simulink model "InvertedPendulum_sim"  (R2019a)
settings: Solver=ode113  StartTime=0.0  StopTime=100  RelTol=1e-3
settings Model: Creator=黄原  LastModifiedBy=黄原

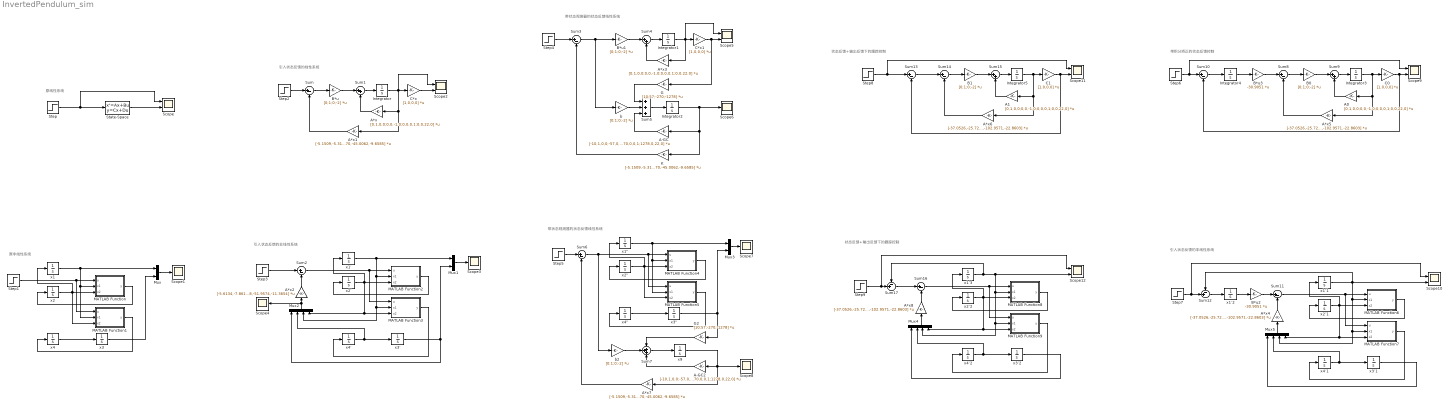
== system InvertedPendulum_sim ==
  note: 原非线性系统
  note: 原线性系统
  note: 引入状态反馈的线性系统
  note: 引入状态反馈的非线性系统
  note: 带状态观测器的状态反馈线性系统
  note: 带状态观测器的状态反馈线性系统
  note: 带积分矫正的状态反馈控制
  note: 引入状态反馈的非线性系统
  note: 状态反馈+输出反馈下的跟踪控制
  note: 状态反馈+输出反馈下的跟踪控制
  A*x : Gain  Gain=[0,1,0,0;0,0,-1,0;0,0,0,1;0,0,22,0]  Multiplication=Matrix(K*u)
  A*x1 : Gain  Gain=[-5.1509,-5.3170,-45.0062,-9.6585]  Multiplication=Matrix(K*u)
  A*x2 : Gain  Gain=[-5.6134,-7.8618,-51.9574,-11.3654]  Multiplication=Matrix(K*u)
  A*x3 : Gain  Gain=[0,1,0,0;0,0,-1,0;0,0,0,1;0,0,22,0]  Multiplication=Matrix(K*u)
  A*x{4..6,8} (4 alike) : Gain  Gain=[-37.0526,-25.7207,-102.9571,-22.8603]  Multiplication=Matrix(K*u)
  A*x7 : Gain  Gain=[-5.1509,-5.3170,-45.0062,-9.6585]  Multiplication=Matrix(K*u)
  A-GC : Gain  Gain=[-10,1,0,0;-57,0,-1,0;270,0,0,1;1278,0,22,0]  Multiplication=Matrix(K*u)
  A-GC2 : Gain  Gain=[-10,1,0,0;-57,0,-1,0;270,0,0,1;1278,0,22,0]  Multiplication=Matrix(K*u)
  A0 : Gain  Gain=[0,1,0,0;0,0,-1,0;0,0,0,1;0,0,22,0]  Multiplication=Matrix(K*u)
  A1 : Gain  Gain=[0,1,0,0;0,0,-1,0;0,0,0,1;0,0,22,0]  Multiplication=Matrix(K*u)
  B*u : Gain  Gain=[0;1;0;-2]  Multiplication=Matrix(K*u)
  B*u1 : Gain  Gain=[0;1;0;-2]  Multiplication=Matrix(K*u)
  B*u2 : Gain  Gain=-30.9051  Multiplication=Matrix(K*u)
  B*u3 : Gain  Gain=-30.9051  Multiplication=Matrix(K*u)
  B0 : Gain  Gain=[0;1;0;-2]  Multiplication=Matrix(K*u)
  B1 : Gain  Gain=[0;1;0;-2]  Multiplication=Matrix(K*u)
  C*x : Gain  Gain=[1,0,0,0]  Multiplication=Matrix(K*u)
  C*x1 : Gain  Gain=[1,0,0,0]  Multiplication=Matrix(K*u)
  C0 : Gain  Gain=[1,0,0,0]  Multiplication=Matrix(K*u)
  C1 : Gain  Gain=[1,0,0,0]  Multiplication=Matrix(K*u)
  G : Gain  Gain=[10;57;-270;-1278]  Multiplication=Matrix(K*u)
  G2 : Gain  Gain=[10;57;-270;-1278]  Multiplication=Matrix(K*u)
  Integrator{,1..2,5} (4 alike) : Integrator  InitialCondition=[0.1,0.1,0.1,0.1]
  Integrator3 : Integrator  InitialCondition=[0,0,0,0]
  Integrator4 : Integrator
  K : Gain  Gain=[-5.1509,-5.3170,-45.0062,-9.6585]  Multiplication=Matrix(K*u)
  MATLAB Function : MATLAB Function  TreatAsAtomicUnit=on
  MATLAB Function1 : MATLAB Function  TreatAsAtomicUnit=on
  MATLAB Function2 : MATLAB Function  TreatAsAtomicUnit=on
  MATLAB Function3 : MATLAB Function  TreatAsAtomicUnit=on
  MATLAB Function4 : MATLAB Function  TreatAsAtomicUnit=on
  MATLAB Function5 : MATLAB Function  TreatAsAtomicUnit=on
  MATLAB Function6 : MATLAB Function  TreatAsAtomicUnit=on
  MATLAB Function7 : MATLAB Function  TreatAsAtomicUnit=on
  MATLAB Function8 : MATLAB Function  TreatAsAtomicUnit=on
  MATLAB Function9 : MATLAB Function  TreatAsAtomicUnit=on
  Mux : Mux  Inputs=2
  Mux1 : Mux  Inputs=2
  Mux2 : Mux
  Mux3 : Mux  Inputs=2
  Mux4 : Mux
  Mux5 : Mux
  Scope{,2,5,9..12} (7 alike) : Scope  NumInputPorts=2
  Scope{1,3..4,6..8} (6 alike) : Scope
  State-Space : StateSpace  A=[0,1,0,0;0,0,-1,0;0,0,0,1;0,0,22,0]  B=[0;1;0;-2]  C=[1,0,0,0]  D=0  InitialCondition=[0.1;0.1;0.1;0.1]
  Step{,1..5} (6 alike) : Step  After=0.01  SampleTime=0
  Step6 : Step  Time=3  SampleTime=0
  Step7 : Step  After=0.05  SampleTime=0
  Step8 : Step  After=0.05  SampleTime=0
  Step9 : Step  After=0.05  SampleTime=0
  Sum{,2..3,6,8,10..11,13..14,16} (10 alike) : Sum  Inputs=|+-
  Sum{1,4,9,15} (4 alike) : Sum  Inputs=|++
  Sum12 : Sum  Inputs=-+|
  Sum17 : Sum  Inputs=-+|
  Sum5 : Sum  Inputs=+++
  Sum7 : Sum  Inputs=+++
  b : Gain  Gain=[0;1;0;-2]  Multiplication=Matrix(K*u)
  b2 : Gain  Gain=[0;1;0;-2]  Multiplication=Matrix(K*u)
  x{1..4,9} (5 alike) : Integrator  InitialCondition=0.1
  x1'' : Integrator  InitialCondition=0.1
  x1‘ : Integrator  InitialCondition=0.1
  x1‘1 : Integrator  InitialCondition=0.1
  x1‘2 : Integrator
  x1‘3 : Integrator  InitialCondition=0.1
  "x2'' " : Integrator  InitialCondition=0.1
  x2’ : Integrator  InitialCondition=0.1
  x2’1 : Integrator  InitialCondition=0.1
  x2’2 : Integrator  InitialCondition=0.1
  x3'' : Integrator  InitialCondition=0.1
  x3’ : Integrator  InitialCondition=0.1
  x3’1 : Integrator  InitialCondition=0.1
  x3’2 : Integrator  InitialCondition=0.1
  x4'' : Integrator  InitialCondition=0.1
  x4‘ : Integrator  InitialCondition=0.1
  x4‘1 : Integrator  InitialCondition=0.1
  x4‘2 : Integrator  InitialCondition=0.1
  wires:
  x1/1 -> MATLAB Function1/2(x1), MATLAB Function/2(x1), Mux/1
  x2/1 -> x1/1, MATLAB Function/3(x2), MATLAB Function1/3(x2)
  MATLAB Function/1(y) -> x2/1
  x4/1 -> x3/1
  MATLAB Function1/1(y) -> x4/1
  Mux/1 -> Scope1/1
  x3/1 -> Mux/2
  State-Space/1 -> Scope/2
  Step1/1 -> MATLAB Function1/1(u), MATLAB Function/1(u)
  Step/1 -> State-Space/1, Scope/1
  Step2/1 -> Sum/1
  Sum/1 -> B*u/1
  B*u/1 -> Sum1/1
  Sum1/1 -> Integrator/1
  A*x/1 -> Sum1/2
  Integrator/1 -> A*x1/1, A*x/1, Scope2/1, C*x/1
  C*x/1 -> Scope2/2
  A*x1/1 -> Sum/2
  x1‘/1 -> Mux2/3, MATLAB Function3/2(x1), MATLAB Function2/2(x1), Mux1/1
  MATLAB Function2/1(y) -> x2’/1
  x2’/1 -> MATLAB Function2/3(x2), x1‘/1, Mux2/4, MATLAB Function3/3(x2)
  MATLAB Function3/1(y) -> x4‘/1
  Mux1/1 -> Scope3/1
  x3’/1 -> Mux1/2, Mux2/1
  x4‘/1 -> Mux2/2, x3’/1
  Step3/1 -> Sum2/1
  Sum2/1 -> MATLAB Function2/1(u), MATLAB Function3/1(u)
  A*x2/1 -> Sum2/2
  Mux2/1 -> Scope4/1, A*x2/1
  C*x1/1 -> G/1, Scope5/2
  Sum3/1 -> b/1, B*u1/1
  Sum4/1 -> Integrator1/1
  Integrator1/1 -> A*x3/1, Scope5/1, C*x1/1
  B*u1/1 -> Sum4/1
  Step4/1 -> Sum3/1
  A*x3/1 -> Sum4/2
  b/1 -> Sum5/2
  G/1 -> Sum5/1
  Sum5/1 -> Integrator2/1
  Integrator2/1 -> K/1, A-GC/1, Scope6/1
  A-GC/1 -> Sum5/3
  K/1 -> Sum3/2
  x1''/1 -> MATLAB Function5/2(x1), MATLAB Function4/2(x1), Mux3/1
  MATLAB Function4/1(y) -> "x2'' "/1
  "x2'' "/1 -> x1''/1, MATLAB Function4/3(x2), MATLAB Function5/3(x2)
  MATLAB Function5/1(y) -> x4''/1
  Mux3/1 -> Scope7/1
  x3''/1 -> G2/1, Mux3/2
  x4''/1 -> x3''/1
  Step5/1 -> Sum6/1
  Sum6/1 -> MATLAB Function5/1(u), MATLAB Function4/1(u), b2/1
  b2/1 -> Sum7/2
  Sum7/1 -> x9/1
  G2/1 -> Sum7/1
  A-GC2/1 -> Sum7/3
  x9/1 -> Scope8/1, A*x7/1, A-GC2/1
  A*x7/1 -> Sum6/2
  C0/1 -> Sum10/2, Scope9/2
  Sum8/1 -> B0/1
  A*x5/1 -> Sum8/2
  Sum9/1 -> Integrator3/1
  Integrator3/1 -> A*x5/1, A0/1, C0/1
  B0/1 -> Sum9/1
  A0/1 -> Sum9/2
  B*u3/1 -> Sum8/1
  Integrator4/1 -> B*u3/1
  Sum10/1 -> Integrator4/1
  Step6/1 -> Sum10/1, Scope9/1
  Sum11/1 -> MATLAB Function6/1(u), MATLAB Function7/1(u)
  A*x4/1 -> Sum11/2
  x4‘1/1 -> Mux5/2, x3’1/1
  x3’1/1 -> Mux5/1
  x1‘1/1 -> Scope10/2, Sum12/1, Mux5/3, MATLAB Function7/2(x1), MATLAB Function6/2(x1)
  MATLAB Function6/1(y) -> x2’1/1
  x2’1/1 -> MATLAB Function6/3(x2), x1‘1/1, Mux5/4, MATLAB Function7/3(x2)
  Mux5/1 -> A*x4/1
  MATLAB Function7/1(y) -> x4‘1/1
  Step7/1 -> Sum12/2, Scope10/1
  Sum12/1 -> x1‘2/1
  x1‘2/1 -> B*u2/1
  B*u2/1 -> Sum11/1
  Sum13/1 -> Sum14/1
  A1/1 -> Sum15/2
  Integrator5/1 -> A*x6/1, A1/1, C1/1
  C1/1 -> Sum13/2, Scope11/2
  Sum14/1 -> B1/1
  B1/1 -> Sum15/1
  Sum15/1 -> Integrator5/1
  Step8/1 -> Sum13/1, Scope11/1
  A*x6/1 -> Sum14/2
  Sum17/1 -> Sum16/1
  Mux4/1 -> A*x8/1
  MATLAB Function9/1(y) -> x4‘2/1
  x2’2/1 -> MATLAB Function8/3(x2), x1‘3/1, Mux4/4, MATLAB Function9/3(x2)
  x1‘3/1 -> Scope12/2, Mux4/3, MATLAB Function9/2(x1), MATLAB Function8/2(x1), Sum17/1
  MATLAB Function8/1(y) -> x2’2/1
  x4‘2/1 -> Mux4/2, x3’2/1
  x3’2/1 -> Mux4/1
  A*x8/1 -> Sum16/2
  Step9/1 -> Scope12/1, Sum17/2
  Sum16/1 -> MATLAB Function8/1(u), MATLAB Function9/1(u)

== matlab function InvertedPendulum_sim/MATLAB Function1 ==
  data: u input; y output; x1 input; x2 input
function y = fcn(u,x1,x2)

y = (u+0.05*sin(x1*x2*x2)-cos(x1)*sin(x1))/(1.1-0.1*cos(x1)*cos(x1));

== matlab function InvertedPendulum_sim/MATLAB Function ==
  data: u input; y output; x1 input; x2 input
function y = fcn(u,x1,x2)

y = (u*cos(x1)-11*sin(x1)+0.05*sin(x1)*cos(x1)*x2*x2)/(0.05*cos(x1)*cos(x1)-0.55);

== matlab function InvertedPendulum_sim/MATLAB Function2 ==
  data: u input; y output; x1 input; x2 input
function y = fcn(u, x1, x2)

y = (u*cos(x1)-11*sin(x1)+0.05*sin(x1)*cos(x1*x2*x2))/(0.05*cos(x1)*cos(x1)-0.55);

== matlab function InvertedPendulum_sim/MATLAB Function3 ==
  data: u input; y output; x1 input; x2 input
function y = fcn(u, x1, x2)

y = (u+0.05*sin(x1*x2*x2)-cos(x1)*sin(x1))/(1.1-0.1*cos(x1)*cos(x1));

== matlab function InvertedPendulum_sim/MATLAB Function4 ==
  data: u input; y output; x1 input; x2 input
function y = fcn(u,x1,x2)

y = (u*cos(x1)-11*sin(x1)+0.05*sin(x1)*cos(x1)*x2*x2)/(0.05*cos(x1)*cos(x1)-0.55);

== matlab function InvertedPendulum_sim/MATLAB Function5 ==
  data: u input; y output; x1 input; x2 input
function y = fcn(u,x1,x2)

y = (u+0.05*sin(x1)*x2*x2-cos(x1)*sin(x1))/(1.1-0.1*cos(x1)*cos(x1));

== matlab function InvertedPendulum_sim/MATLAB Function6 ==
  data: u input; y output; x1 input; x2 input
function y = fcn(u, x1, x2)

y = (u*cos(x1)-11*sin(x1)+0.05*sin(x1)*cos(x1)*x2*x2)/(0.05*cos(x1)*cos(x1)-0.55);

== matlab function InvertedPendulum_sim/MATLAB Function7 ==
  data: u input; y output; x1 input; x2 input
function y = fcn(u, x1, x2)

y = (u+0.05*sin(x1)*x2*x2-cos(x1)*sin(x1))/(1.1-0.1*cos(x1)*cos(x1));

== matlab function InvertedPendulum_sim/MATLAB Function8 ==
  data: u input; y output; x1 input; x2 input
function y = fcn(u, x1, x2)

y = (u*cos(x1)-11*sin(x1)+0.05*sin(x1)*cos(x1*x2*x2))/(0.05*cos(x1)*cos(x1)-0.55);

== matlab function InvertedPendulum_sim/MATLAB Function9 ==
  data: u input; y output; x1 input; x2 input
function y = fcn(u, x1, x2)

y = (u+0.05*sin(x1*x2*x2)-cos(x1)*sin(x1))/(1.1-0.1*cos(x1)*cos(x1));
